simulink model "Simulacion"  (R2022b)
settings: Solver=ode1be  StartTime=0.0  StopTime=100  FixedStep=h  RelTol=1e-3
values from neighbouring files (symbols this model uses):
  A = A + size * eye(size)    [IniciadorParametros.m]
  B = [zeros(nq,m) ... (first row only)    [IniciadorParametros.m]
  h = 0.01    [IniciadorParametros.m]
  K1 = 2.2802    [IniciadorParametros.m]
  K2 = 2.7468    [IniciadorParametros.m]
  nq = dof*(nn-nbc)    [IniciadorParametros.m]
  P = I    (= 4.21875e-13)    [IniciadorParametros.m]
  V0 = V1    [IniciadorParametros.m]
  W0 = W1    [IniciadorParametros.m]
undefined symbols (not defined in the file or in its folder): f
settings Model: Creator=raul  LastModifiedBy=raul

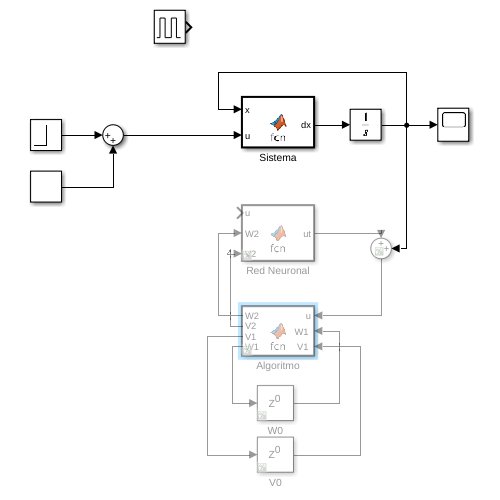
[thumbnail: Simulink's stored preview of the top-level diagram]
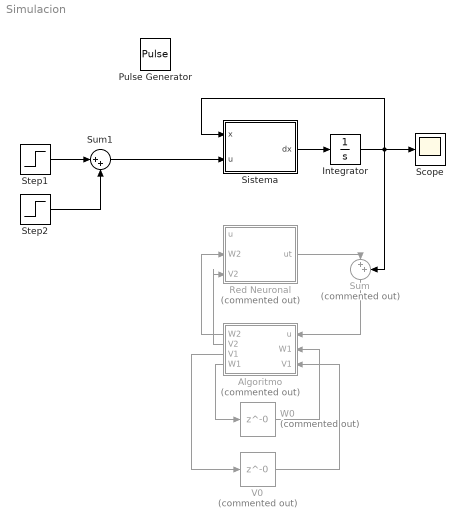
== system Simulacion ==
  Algoritmo : MATLAB Function  Commented=on  TreatAsAtomicUnit=on
  Integrator : Integrator  InitialCondition=zeros(2*nq,1)
  Pulse Generator : DiscretePulseGenerator  PulseType=Time based  Period=1  PulseWidth=5
  Red Neuronal : MATLAB Function  Commented=on  TreatAsAtomicUnit=on
  Scope : Scope
  Sistema : MATLAB Function  TreatAsAtomicUnit=on
  Step1 : Step  SampleTime=0
  Step2 : Step  Time=1.1  After=-1  SampleTime=0
  Sum : Sum  Commented=on  Inputs=|++
  Sum1 : Sum  Inputs=|++
  V0 : Delay  Commented=on  DelayLength=0  InitialCondition=V0
  W0 : Delay  Commented=on  DelayLength=0  InitialCondition=W0
  wires:
  Sum/1 -> Algoritmo/1(u)
  Red Neuronal/1(ut) -> Sum/1
  Step2/1 -> Sum1/2
  Step1/1 -> Sum1/1
  Sistema/1(dx) -> Integrator/1
  Integrator/1 -> Scope/1, Sum/2, Sistema/1(x)
  Algoritmo/1(W2) -> Red Neuronal/2(W2)
  W0/1 -> Algoritmo/2("W1 ")
  Algoritmo/2(V2) -> Red Neuronal/3(V2)
  V0/1 -> Algoritmo/3("V1 ")
  Sum1/1 -> Sistema/2(u)
  Algoritmo/4(W1) -> W0/1
  Algoritmo/3(V1) -> V0/1

== matlab function Simulacion/Algoritmo ==
  data: u input; W2 output; V2 output; W1 input; V1 input; f parameter; K1 parameter; K2 parameter; h parameter; P parameter; V1 output; W1 output
function [W2,V2,V1,W1] = fcn(u,W1,V1,f,K1, K2,h,P)

us=1;    %%%%NO se que es realmente "us" preguntar a Rita

[k1u, k1W, k1V] = DNN(u,us,W1,V1,h);

[k2u, k2W, k2V] = DNN(u+.5*k1u,us,W1+.5*k1W,V1+.5*k1V,h);
[k3u, k3W, k3V] = DNN(u+.5*k2u,us,W1+.5*k2W,V1+.5*k2V,h);

[k4u, k4W, k4V] = DNN(u+k3u,us,W1+k3W,V1+k3V,h);

u  =  u + 1/6*k1u + 1/3*k2u + 1/3*k3u + 1/6*k4u;
V1 = V1 + 1/6*k1V + 1/3*k2V + 1/3*k3V + 1/6*k4V;
W1 = W1 + 1/6*k1W + 1/3*k2W + 1/3*k3W + 1/6*k4W;
V2=V1(:,f);  %cambie los valores porque tengo un problema con tamaños de matrices
W2=W1(:,f);  %% lo mismo


function [du, dW, dV] = DNN(u, us, W1, V1, h)
	Delta   = u - us;
	sigma   = sigmoid(1,V1*u);
	D_sigma = diag(sigma.*(1-sigma));
	%
	dW      = h*(-K1*P*Delta*sigma' + K1*P*Delta*u'*(V1-V0)'*D_sigma);
	dV		= h*(-K2*D_sigma'*W1'*P*Delta*u' - l/2*K2*Lambda*(V1-V0)*(u*u'));
	du		= h*(A*u + W1*sigma);
end


function s = sigmoid(b,x)
   s = 1./(1+exp(-b*x)); 
end

end

== matlab function Simulacion/Red Neuronal ==
  data: u input; ut output; A parameter; W2 input; V2 input
function ut = fcn(u,A, W2, V2)

ut = A*u+W2*sigmoid(1,V2*u);


function s = sigmoid(b,x)
   s = 1./(1+exp(-b*x)); 
end

end

== matlab function Simulacion/Sistema ==
  data: x input; u input; dx output; A parameter; B parameter; f parameter
function dx = fcn(x,u,A, B, f)%add Bw,w

dx = A*x+B(:,f)*u;

%dx = A*x+B(:,f)*u+Bw*w;
